simulink model "DUALportRAMinterface_v2"  (R2024a)
settings: Solver=FixedStepDiscrete  StartTime=0.0  StopTime=20  RelTol=1e-3
values from neighbouring files (symbols this model uses):
  Ts = 1/Fs    (= 7.50007500075e-06)    [new_generation_coeff.m]    (also in simon_test.m; simple_fft_test.m = 1/F; testPSD_c2d.m; testPSD_simulink.m)
undefined symbols (not defined in the file or in its folder): magnitude
libraries: hdlsllib x226, embmathops x6, simulink x1, hdlmdlgenlib x1, dsphdlxfrm2 x1
(part 1 of 5)
settings Model: DataTypeOverride=Off  Creator=Simon  LastModifiedBy=Simon
settings OptimizationCC: BlockReduction=off  ConditionallyExecuteInputs=off  DefaultParameterBehavior=Inlined  InheritOutputTypeSmallerThanSingle=on
settings DebuggingCC: AlgebraicLoopMsg=error  SingleTaskRateTransMsg=error  UnconnectedInputMsg=warning  UnconnectedOutputMsg=warning  UnconnectedLineMsg=warning
settings HardwareCC: ProdBitPerPointer=32  ProdBitPerSizeT=32  ProdBitPerPtrDiffT=32  ProdLargestAtomicFloat=None  ProdIntDivRoundTo=Undefined  ProdEndianess=Unspecified  ProdWordSize=32  ProdHWDeviceType=ASIC/FPGA->ASIC/FPGA  TargetBitPerPointer=64  TargetBitPerSizeT=64  TargetBitPerPtrDiffT=64  TargetLongLongMode=on  TargetIntDivRoundTo=Zero  TargetEndianess=LittleEndian  TargetWordSize=64  TargetHWDeviceType=Custom Processor->MATLAB Host Computer  ProdEqTarget=off

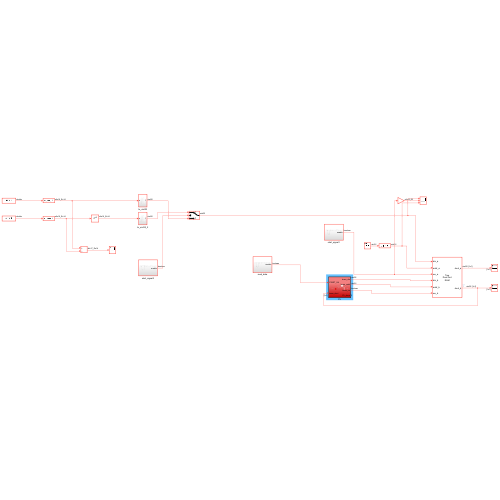
[thumbnail: Simulink's stored preview of the top-level diagram]
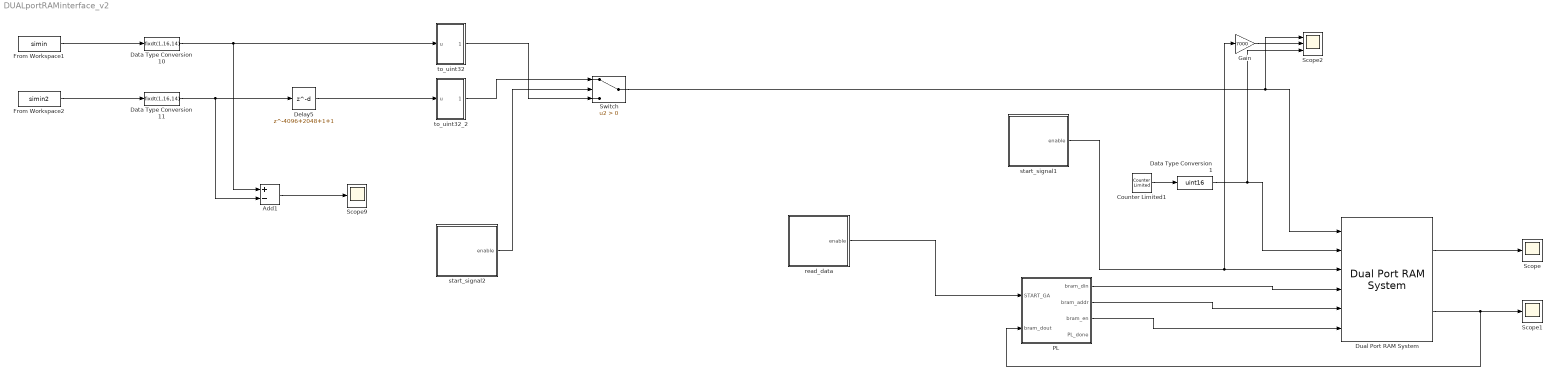
== system DUALportRAMinterface_v2 ==
  Add1 : Sum  Inputs=+-
  Counter Limited1 : simulink/Sources/Counter Limited  uplimit=14000  tsamp=Ts
  Data Type Conversion1 : DataTypeConversion  OutDataTypeStr=uint16  SaturateOnIntegerOverflow=off  RndMeth=Floor
  Data Type Conversion10 : DataTypeConversion  OutDataTypeStr=fixdt(1,16,14)  SaturateOnIntegerOverflow=off  RndMeth=Floor
  Data Type Conversion11 : DataTypeConversion  OutDataTypeStr=fixdt(1,16,14)  SaturateOnIntegerOverflow=off  RndMeth=Floor
  Delay5 : Delay  DelayLength=4096+2048+1+1  InitialCondition=0  SampleTime=Ts
  Dual Port RAM System : hdlsllib/HDL RAMs/Dual Port RAM System  RAMType=True dual port  AsyncRead=off  WriteOutputValue=New data  RAMInitialValue=0  allowBusInputs=off  WritesHaveOutput=on  NumReads=0  NumWrites=1  SimulateUsing=Code generation
  From Workspace1 : FromWorkspace  VariableName=simin  SampleTime=Ts
  From Workspace2 : FromWorkspace  VariableName=simin2  SampleTime=Ts
  Gain : Gain  Gain=7000
  PL : Subsystem
  Scope : Scope
  Scope1 : Scope
  Scope2 : Scope  NumInputPorts=3
  Scope9 : Scope
  Switch : Switch  Criteria=u2 > Threshold  SaturateOnIntegerOverflow=off  InputSameDT=off  OutDataTypeStr=Inherit: Same as first input
  read_data : Subsystem
  start_signal1 : Subsystem
  start_signal2 : Subsystem
  to_uint32 : Subsystem
  to_uint32_2 : Subsystem
  wires:
  Dual Port RAM System/1 -> Scope/1
  Counter Limited1/1 -> Data Type Conversion1/1
  Data Type Conversion1/1 -> Scope2/3, Dual Port RAM System/2
  start_signal1/1(enable) -> Dual Port RAM System/3, Gain/1
  PL/1(bram_din) -> Dual Port RAM System/4
  PL/2(bram_addr) -> Dual Port RAM System/5
  PL/3(bram_en) -> Dual Port RAM System/6
  Gain/1 -> Scope2/2
  read_data/1(enable) -> PL/1(START_GA)
  Dual Port RAM System/2 -> Scope1/1, PL/2(bram_dout)
  From Workspace1/1 -> Data Type Conversion10/1
  From Workspace2/1 -> Data Type Conversion11/1
  to_uint32/1(Out1) -> Switch/3
  to_uint32_2/1(Out1) -> Switch/1
  start_signal2/1(enable) -> Switch/2
  Delay5/1 -> to_uint32_2/1(u)
  Switch/1 -> Scope2/1, Dual Port RAM System/1
  Data Type Conversion11/1 -> Delay5/1, Add1/2
  Add1/1 -> Scope9/1
  Data Type Conversion10/1 -> Add1/1, to_uint32/1(u)

== system DUALportRAMinterface_v2/PL ==
  START_GA : Inport
  bram_dout : Inport  Port=2
  Bit Shift18 : hdlsllib/Logic and Bit Operations/Bit Shift  mode=Shift Right Logical  N=14
  Chart : Stateflow chart  TreatAsAtomicUnit=on
      settings: PortSchema="{\"entries\":[{\"content\":{\"sides\":[{\"content\":{\"connectorIds\":[\"In2\",\"In3\"]},\"type\":\"ConnectorPlacement.EquallySpacedRectSide\",\"uuid\":\"f3ce331f-c708-4668-a9cb-fb327ea74ab5\"},{\"content\":{\"connectorIds\":[\"Out1\",\"Out2\",\"Out3\"],\"side\":\"RIGHT\"},\"type\":\"ConnectorPlacement.EquallySpacedRectSide\",\"uuid\":\"3766927a-abff-497d-9544-2098881ba174\"},{\"content\":{\"side\":\"TOP\"},\"type\":\"ConnectorPlacement.EquallySpacedRectSide\",\"uuid\":\"ebfe3d64-ee7d-4953-a6ba-e7e40988decf\"},{\"content\":{\"connectorIds\":[\"In1\"],\"side\":\"BOTTOM\"},\"type\":\"ConnectorPlacement.EquallySpacedRectSide\",\"uuid\":\"f39ceaf8-4df7-4e40-9de5-da7597831fb4\"}]},\"type\":\"ConnectorPlacement.EquallySpacedConnector\",\"uuid\":\"89f60450-5933-42bb-b72b-5f8ec55483e0\"}],\"packageUris\":[\"http://schema.mathworks.com/mf0/Connector/R2020b\"],\"version\":\"1.0\"}"
  Data Type Conversion2 : DataTypeConversion  OutDataTypeStr=uint32  SaturateOnIntegerOverflow=off  RndMeth=Floor
  Data Type Conversion8 : DataTypeConversion  OutDataTypeStr=fixdt(0,30,14)  SaturateOnIntegerOverflow=off  RndMeth=Floor
  Data Type Conversion9 : DataTypeConversion  OutDataTypeStr=fixdt(1,16,14)  SaturateOnIntegerOverflow=off  RndMeth=Floor
  Delay : Delay  DelayLength=16  InitialCondition=0  SampleTime=Ts
  Demux : Demux  Outputs=7
  Multiport Switch : MultiPortSwitch  DataPortOrder=Specify indices  Inputs=8  DataPortIndices={0,1,2,3,4,5,6,7}  DataPortForDefault=Additional data port  DiagnosticForDefault=None  SaturateOnIntegerOverflow=off  InputSameDT=off
  index_counter : Subsystem
  integration_block1 : Subsystem
  to_uint32_1 : Subsystem
  to_uint32_2 : Subsystem
  to_uint32_3 : Subsystem
  to_uint32_4 : Subsystem
  to_uint32_5 : Subsystem
  to_uint32_6 : Subsystem
  bram_din : Outport
  bram_addr : Outport  Port=2
  bram_en : Outport  Port=3
  PL_done : Outport  Port=4
  wires:
  Multiport Switch/1 -> [PL_data]
  [counter_reset] -> index_counter/2(In2)
  index_counter/1(index_counter) -> Chart/3(counter), [address]
  [address] -> bram_addr/1
  [counter_increment] -> index_counter/1(In1)
  [address] -> Multiport Switch/1
  Chart/3(write_enable) -> [write_enable]
  integration_block1/1(ga_done) -> Delay/1, Chart/1(GA_done)
  START_GA/1 -> Chart/2(GPIO), integration_block1/3(start_ga)
  Chart/2(counter_reset) -> [counter_reset]
  Chart/1(counter_increment) -> [counter_increment]
  [PL_data] -> bram_din/1
  [write_enable] -> bram_en/1
  integration_block1/2(elite_individual) -> Demux/1
  Demux/1 -> Data Type Conversion2/1
  Demux/2 -> to_uint32_1/1(u_port)
  Demux/3 -> to_uint32_2/1(u_port)
  Demux/4 -> to_uint32_3/1(u_port)
  Demux/5 -> to_uint32_4/1(u_port)
  Demux/6 -> to_uint32_5/1(u_port)
  Demux/7 -> to_uint32_6/1(u_port)
  Data Type Conversion2/1 -> Multiport Switch/10, Multiport Switch/9, Multiport Switch/2
  to_uint32_1/1(Out1) -> Multiport Switch/3
  to_uint32_2/1(Out1) -> Multiport Switch/4
  to_uint32_3/1(Out1) -> Multiport Switch/5
  to_uint32_4/1(Out1) -> Multiport Switch/6
  to_uint32_5/1(Out1) -> Multiport Switch/7
  to_uint32_6/1(Out1) -> Multiport Switch/8
  Data Type Conversion9/1 -> integration_block1/1(data_in), integration_block1/2(data_in1)
  Bit Shift18/1 -> Data Type Conversion9/1
  Data Type Conversion8/1 -> Bit Shift18/1
  bram_dout/1 -> Data Type Conversion8/1
  [PL_done] -> PL_done/1
  Delay/1 -> [PL_done]

== system DUALportRAMinterface_v2/read_data ==
  Data Type Conversion29 : DataTypeConversion  OutDataTypeStr=boolean  SaturateOnIntegerOverflow=off  RndMeth=Floor
  Delay2 : Delay  DelayLength=1  InitialCondition=0  SampleTime=Ts
  Gain : Gain
  Step1 : Step  Time=Ts*14000  SampleTime=Ts
  XOR1 : Logic  Operator=XOR  IconShape=distinctive  AllPortsSameDT=off  OutDataTypeStr=boolean
  enable : Outport
  wires:
  XOR1/1 -> Gain/1
  Step1/1 -> Delay2/1, XOR1/1
  Delay2/1 -> XOR1/2
  Gain/1 -> Data Type Conversion29/1
  Data Type Conversion29/1 -> enable/1

== system DUALportRAMinterface_v2/start_signal1 ==
  Data Type Conversion29 : DataTypeConversion  OutDataTypeStr=boolean  SaturateOnIntegerOverflow=off  RndMeth=Floor
  Delay2 : Delay  DelayLength=(4096+2048+1+1)*2  InitialCondition=0  SampleTime=Ts
  Gain : Gain
  Step1 : Step  Time=Ts*0  SampleTime=Ts
  XOR1 : Logic  Operator=XOR  IconShape=distinctive  AllPortsSameDT=off  OutDataTypeStr=boolean
  enable : Outport
  wires:
  Data Type Conversion29/1 -> enable/1
  Gain/1 -> Data Type Conversion29/1
  Delay2/1 -> XOR1/2
  Step1/1 -> XOR1/1, Delay2/1
  XOR1/1 -> Gain/1

== system DUALportRAMinterface_v2/start_signal2 ==
  Data Type Conversion29 : DataTypeConversion  OutDataTypeStr=boolean  SaturateOnIntegerOverflow=off  RndMeth=Floor
  Delay2 : Delay  DelayLength=(4096+2048+1+1)*2  InitialCondition=0  SampleTime=Ts
  Gain : Gain
  Step1 : Step  Time=Ts*(4096+2048+1+1)  SampleTime=Ts
  XOR1 : Logic  Operator=XOR  IconShape=distinctive  AllPortsSameDT=off  OutDataTypeStr=boolean
  enable : Outport
  wires:
  XOR1/1 -> Gain/1
  Step1/1 -> Delay2/1, XOR1/1
  Delay2/1 -> XOR1/2
  Gain/1 -> Data Type Conversion29/1
  Data Type Conversion29/1 -> enable/1

== system DUALportRAMinterface_v2/to_uint32 ==
  u : Inport
  Bit Concat2 : hdlsllib/Logic and Bit Operations/Bit Concat  numInputs=16
  Bit Shift19 : hdlsllib/Logic and Bit Operations/Bit Shift  mode=Shift Left Logical  N=1
  Bit Shift20 : hdlsllib/Logic and Bit Operations/Bit Shift  mode=Shift Left Logical  N=10
  Bit Shift21 : hdlsllib/Logic and Bit Operations/Bit Shift  mode=Shift Right Logical  N=1
  Bit Shift22 : hdlsllib/Logic and Bit Operations/Bit Shift  mode=Shift Left Logical  N=11
  Bit Shift23 : hdlsllib/Logic and Bit Operations/Bit Shift  mode=Shift Left Logical  N=12
  Bit Shift24 : hdlsllib/Logic and Bit Operations/Bit Shift  mode=Shift Left Logical  N=13
  Bit Shift25 : hdlsllib/Logic and Bit Operations/Bit Shift  mode=Shift Left Logical  N=14
  Bit Shift26 : hdlsllib/Logic and Bit Operations/Bit Shift  mode=Shift Left Logical  N=2
  Bit Shift27 : hdlsllib/Logic and Bit Operations/Bit Shift  mode=Shift Left Logical  N=3
  Bit Shift28 : hdlsllib/Logic and Bit Operations/Bit Shift  mode=Shift Left Logical  N=4
  Bit Shift29 : hdlsllib/Logic and Bit Operations/Bit Shift  mode=Shift Left Logical  N=5
  Bit Shift30 : hdlsllib/Logic and Bit Operations/Bit Shift  mode=Shift Left Logical  N=6
  Bit Shift31 : hdlsllib/Logic and Bit Operations/Bit Shift  mode=Shift Left Logical  N=7
  Bit Shift32 : hdlsllib/Logic and Bit Operations/Bit Shift  mode=Shift Left Logical  N=8
  Bit Shift33 : hdlsllib/Logic and Bit Operations/Bit Shift  mode=Shift Left Logical  N=9
  Data Type Conversion{12..16,26,34..43} (16 alike) : DataTypeConversion  OutDataTypeStr=fixdt(0,1,0)  SaturateOnIntegerOverflow=off  RndMeth=Floor
  Data Type Conversion44 : DataTypeConversion  OutDataTypeStr=uint32  SaturateOnIntegerOverflow=off  RndMeth=Floor
  Out1 : Outport
  wires:
  Bit Shift22/1 -> Data Type Conversion40/1
  Bit Shift27/1 -> Data Type Conversion34/1
  Data Type Conversion36/1 -> Bit Concat2/3
  u/1 -> Bit Shift21/1, Data Type Conversion12/1, Bit Shift19/1, Bit Shift26/1, Bit Shift27/1, Bit Shift28/1, Bit Shift29/1, Bit Shift30/1, Bit Shift31/1, Bit Shift32/1, Bit Shift33/1, Bit Shift20/1, Bit Shift22/1, Bit Shift23/1, Bit Shift24/1, Bit Shift25/1
  Bit Shift20/1 -> Data Type Conversion41/1
  Data Type Conversion13/1 -> Bit Concat2/1
  Data Type Conversion40/1 -> Bit Concat2/13
  Bit Shift31/1 -> Data Type Conversion43/1
  Data Type Conversion26/1 -> Bit Concat2/6
  Data Type Conversion44/1 -> Out1/1
  Data Type Conversion35/1 -> Bit Concat2/4
  Data Type Conversion42/1 -> Bit Concat2/11
  Bit Shift19/1 -> Data Type Conversion36/1
  Data Type Conversion38/1 -> Bit Concat2/15
  Bit Shift25/1 -> Data Type Conversion37/1
  Data Type Conversion15/1 -> Bit Concat2/8
  Bit Shift30/1 -> Data Type Conversion15/1
  Data Type Conversion12/1 -> Bit Concat2/2
  Bit Shift32/1 -> Data Type Conversion14/1
  Data Type Conversion39/1 -> Bit Concat2/14
  Data Type Conversion34/1 -> Bit Concat2/5
  Data Type Conversion43/1 -> Bit Concat2/9
  Data Type Conversion16/1 -> Bit Concat2/7
  Bit Shift33/1 -> Data Type Conversion42/1
  Bit Shift24/1 -> Data Type Conversion38/1
  Data Type Conversion41/1 -> Bit Concat2/12
  Bit Shift23/1 -> Data Type Conversion39/1
  Bit Shift29/1 -> Data Type Conversion16/1
  Data Type Conversion37/1 -> Bit Concat2/16
  Bit Shift28/1 -> Data Type Conversion26/1
  Bit Shift21/1 -> Data Type Conversion13/1
  Bit Shift26/1 -> Data Type Conversion35/1
  Bit Concat2/1 -> Data Type Conversion44/1
  Data Type Conversion14/1 -> Bit Concat2/10

== system DUALportRAMinterface_v2/to_uint32_2 ==
  u : Inport
  Bit Concat2 : hdlsllib/Logic and Bit Operations/Bit Concat  numInputs=16
  Bit Shift19 : hdlsllib/Logic and Bit Operations/Bit Shift  mode=Shift Left Logical  N=1
  Bit Shift20 : hdlsllib/Logic and Bit Operations/Bit Shift  mode=Shift Left Logical  N=10
  Bit Shift21 : hdlsllib/Logic and Bit Operations/Bit Shift  mode=Shift Right Logical  N=1
  Bit Shift22 : hdlsllib/Logic and Bit Operations/Bit Shift  mode=Shift Left Logical  N=11
  Bit Shift23 : hdlsllib/Logic and Bit Operations/Bit Shift  mode=Shift Left Logical  N=12
  Bit Shift24 : hdlsllib/Logic and Bit Operations/Bit Shift  mode=Shift Left Logical  N=13
  Bit Shift25 : hdlsllib/Logic and Bit Operations/Bit Shift  mode=Shift Left Logical  N=14
  Bit Shift26 : hdlsllib/Logic and Bit Operations/Bit Shift  mode=Shift Left Logical  N=2
  Bit Shift27 : hdlsllib/Logic and Bit Operations/Bit Shift  mode=Shift Left Logical  N=3
  Bit Shift28 : hdlsllib/Logic and Bit Operations/Bit Shift  mode=Shift Left Logical  N=4
  Bit Shift29 : hdlsllib/Logic and Bit Operations/Bit Shift  mode=Shift Left Logical  N=5
  Bit Shift30 : hdlsllib/Logic and Bit Operations/Bit Shift  mode=Shift Left Logical  N=6
  Bit Shift31 : hdlsllib/Logic and Bit Operations/Bit Shift  mode=Shift Left Logical  N=7
  Bit Shift32 : hdlsllib/Logic and Bit Operations/Bit Shift  mode=Shift Left Logical  N=8
  Bit Shift33 : hdlsllib/Logic and Bit Operations/Bit Shift  mode=Shift Left Logical  N=9
  Data Type Conversion{12..16,26,34..43} (16 alike) : DataTypeConversion  OutDataTypeStr=fixdt(0,1,0)  SaturateOnIntegerOverflow=off  RndMeth=Floor
  Data Type Conversion44 : DataTypeConversion  OutDataTypeStr=uint32  SaturateOnIntegerOverflow=off  RndMeth=Floor
  Out1 : Outport
  wires:
  Data Type Conversion14/1 -> Bit Concat2/10
  Bit Concat2/1 -> Data Type Conversion44/1
  Bit Shift26/1 -> Data Type Conversion35/1
  Bit Shift21/1 -> Data Type Conversion13/1
  Bit Shift28/1 -> Data Type Conversion26/1
  Data Type Conversion37/1 -> Bit Concat2/16
  Bit Shift29/1 -> Data Type Conversion16/1
  Bit Shift23/1 -> Data Type Conversion39/1
  Data Type Conversion41/1 -> Bit Concat2/12
  Bit Shift24/1 -> Data Type Conversion38/1
  Bit Shift33/1 -> Data Type Conversion42/1
  Data Type Conversion16/1 -> Bit Concat2/7
  Data Type Conversion43/1 -> Bit Concat2/9
  Data Type Conversion34/1 -> Bit Concat2/5
  Data Type Conversion39/1 -> Bit Concat2/14
  Bit Shift32/1 -> Data Type Conversion14/1
  Data Type Conversion12/1 -> Bit Concat2/2
  Bit Shift30/1 -> Data Type Conversion15/1
  Data Type Conversion15/1 -> Bit Concat2/8
  Bit Shift25/1 -> Data Type Conversion37/1
  Data Type Conversion38/1 -> Bit Concat2/15
  Bit Shift19/1 -> Data Type Conversion36/1
  Data Type Conversion42/1 -> Bit Concat2/11
  Data Type Conversion35/1 -> Bit Concat2/4
  Data Type Conversion44/1 -> Out1/1
  Data Type Conversion26/1 -> Bit Concat2/6
  Bit Shift31/1 -> Data Type Conversion43/1
  Data Type Conversion40/1 -> Bit Concat2/13
  Data Type Conversion13/1 -> Bit Concat2/1
  Bit Shift20/1 -> Data Type Conversion41/1
  u/1 -> Bit Shift25/1, Bit Shift24/1, Bit Shift23/1, Bit Shift22/1, Bit Shift20/1, Bit Shift33/1, Bit Shift32/1, Bit Shift31/1, Bit Shift30/1, Bit Shift29/1, Bit Shift28/1, Bit Shift27/1, Bit Shift26/1, Bit Shift19/1, Data Type Conversion12/1, Bit Shift21/1
  Data Type Conversion36/1 -> Bit Concat2/3
  Bit Shift27/1 -> Data Type Conversion34/1
  Bit Shift22/1 -> Data Type Conversion40/1

== system DUALportRAMinterface_v2/PL/index_counter ==
  In1 : Inport
  In2 : Inport  Port=2
  Add : Sum  OutDataTypeStr=Inherit: Same as first input
  Constant18 : Constant  OutDataTypeStr=fixdt(0,16,0)  SampleTime=Ts
  Constant19 : Constant  Value=0  OutDataTypeStr=fixdt(0,16,0)  SampleTime=Ts
  Constant20 : Constant  Value=0  OutDataTypeStr=uint16  SampleTime=Ts
  Delay : Delay  DelayLength=1  InitialCondition=0  SampleTime=Ts
  Switch : Switch  Criteria=u2 > Threshold  SaturateOnIntegerOverflow=off  InputSameDT=off  OutDataTypeStr=Inherit: Same as first input
  Switch8 : Switch  Criteria=u2 > Threshold  SaturateOnIntegerOverflow=off  InputSameDT=off  OutDataTypeStr=Inherit: Same as first input
  index_counter : Outport
  wires:
  Constant19/1 -> Switch/3
  Switch8/1 -> Add/2
  Switch/1 -> Add/1
  Delay/1 -> index_counter/1, Switch8/3
  In2/1 -> Switch8/2
  Add/1 -> Delay/1
  Constant20/1 -> Switch8/1
  Constant18/1 -> Switch/1
  In1/1 -> Switch/2

== system DUALportRAMinterface_v2/PL/integration_block1 ==
  data_in : Inport
  data_in1 : Inport  Port=2
  start_ga : Inport  Port=3
  D2 : Subsystem
      settings: PortSchema="{\"entries\":[{\"content\":{\"sides\":[{\"content\":{\"connectorIds\":[\"In1\",\"In2\"]},\"type\":\"ConnectorPlacement.EquallySpacedRectSide\",\"uuid\":\"5abe48ab-1b34-4cb0-8d41-07cb17904e64\"},{\"content\":{\"connectorIds\":[\"Out1\"],\"side\":\"RIGHT\"},\"type\":\"ConnectorPlacement.EquallySpacedRectSide\",\"uuid\":\"19bc24ff-88f3-42df-af8e-ecb9c1c6119c\"},{\"content\":{\"connectorIds\":[\"In3\"],\"side\":\"TOP\"},\"type\":\"ConnectorPlacement.EquallySpacedRectSide\",\"uuid\":\"46fc65c4-6cee-4e0a-9107-9d106d0a52a5\"},{\"content\":{\"connectorIds\":[\"In4\"],\"side\":\"BOTTOM\"},\"type\":\"ConnectorPlacement.EquallySpacedRectSide\",\"uuid\":\"10a5fc09-3948-4556-8b0c-050853396926\"}]},\"type\":\"ConnectorPlacement.EquallySpacedConnector\",\"uuid\":\"9cc35bfe-5b00-42b0-9811-425d4f0f8f7b\"}],\"packageUris\":[\"http://schema.mathworks.com/mf0/Connector/R2020b\"],\"version\":\"1.0\"}"
  Delay : Delay  DelayLength=6145  InitialCondition=0  UseCircularBuffer=on  SampleTime=Ts
  Delay3 : Delay  DelayLength=1  InitialCondition=0  SampleTime=Ts
  FFT : dsphdlxfrm2/FFT  Architecture=Burst Radix 2  FFTLengthSource=Property  FFTLength=4096  FFTLengthMax=1024  ComplexMultiplication=Use 4 multipliers and 2 adders  BitReversedOutput=off  BitReversedInput=off  Normalize=off  SimulateUsing=Code generation  RoundingMethod=Floor  ResetInputPort=on  StartOutputPort=off  EndOutputPort=off
  FIFO_system1 : Subsystem
  FIFO_system3 : Subsystem
  GA_main : Subsystem
      settings: PortSchema="{\"entries\":[{\"content\":{\"sides\":[{\"content\":{\"connectorIds\":[\"In1\",\"In2\",\"In3\",\"In4\",\"In5\",\"In6\",\"In7\",\"In8\",\"In9\",\"In10\",\"In11\"]},\"type\":\"ConnectorPlacement.EquallySpacedRectSide\",\"uuid\":\"daccc056-a93f-45e5-9369-71b73e32651e\"},{\"content\":{\"connectorIds\":[\"Out1\",\"Out2\"],\"side\":\"RIGHT\"},\"type\":\"ConnectorPlacement.EquallySpacedRectSide\",\"uuid\":\"82109161-9ebe-455f-914b-56f9927b10eb\"},{\"content\":{\"connectorIds\":[\"Out3\",\"Out4\",\"Out5\",\"In12\",\"In13\"],\"side\":\"TOP\"},\"type\":\"ConnectorPlacement.EquallySpacedRectSide\",\"uuid\":\"07b2e20b-bb92-4769-b746-3d44a115cdd8\"}]},\"type\":\"ConnectorPlacement.EquallySpacedConnector\",\"uuid\":\"c9f522d4-4f80-4900-b8a5-3110692e6ae8\"}],\"packageUris\":[\"http://schema.mathworks.com/mf0/Connector/R2020b\"],\"version\":\"1.0\"}"
  Scope1 : Scope
  Subsystem : Subsystem
  Sum : Sum  Inputs=|+-  OutDataTypeStr=Inherit: Same as first input
  Terminator : Terminator
  Terminator1 : Terminator
  Terminator2 : Terminator
  accumulator_scorer : Subsystem
  ga_done : Outport
  elite_individual : Outport  Port=2
  wires:
  FFT/2 -> accumulator_scorer/2(valid_fft)
  FIFO_system3/2(data_valid) -> Terminator1/1
  accumulator_scorer/1(individual_score) -> GA_main/2(score_result), Scope1/1
  FIFO_system1/1(data_out) -> Sum/1
  start_ga/1 -> GA_main/1(start_ga), Subsystem/1(enable)
  D2/1(response) -> Sum/2
  FFT/1 -> accumulator_scorer/1(data_in)
  FFT/3 -> Terminator/1
  GA_main/5(load_fifo) -> FIFO_system1/3(load_fifo)
  GA_main/4(FIFO_out_en) -> D2/2(push_individual), FIFO_system3/2(enable_output), FIFO_system1/2(enable_output)
  data_in/1 -> FIFO_system1/1(data_in)
  GA_main/2(ga_done) -> ga_done/1
  FIFO_system3/1(data_out) -> D2/1(GAerror)
  GA_main/3(individual_to_d2) -> D2/4(Individual_input)
  accumulator_scorer/2(individual_score_valid) -> Delay3/1
  FIFO_system3/3(reset_fft) -> Terminator2/1
  Delay3/1 -> GA_main/13(score_done)
  data_in1/1 -> FIFO_system3/1(data_in)
  FIFO_system1/2(data_valid) -> FFT/2
  FIFO_system1/3(reset_fft) -> Delay/1, FFT/3
  FIFO_system3/4(FIFO_full) -> GA_main/12(FIFO_full)
  Sum/1 -> FFT/1
  Delay/1 -> D2/3(reset_D2)
  Subsystem/1(random_gene_out) -> GA_main/3(random_gene)
  Subsystem/2(random_method_out) -> GA_main/4(random_method)
  Subsystem/3(b2_random_out) -> GA_main/5(b2rnd)
  Subsystem/4(b3_random_out) -> GA_main/6(b3rnd)
  Subsystem/5(b4_random_out) -> GA_main/7(b4rnd)
  Subsystem/6(a2_random_out) -> GA_main/8(a2rnd)
  Subsystem/7(a3_random_out) -> GA_main/9(a3rnd)
  Subsystem/8(a4_random_out) -> GA_main/10(a4rnd)
  Subsystem/9(random_sample_out) -> GA_main/11(tb_random_sample)
  FIFO_system1/4(FIFO_full) -> FIFO_system3/3(load_fifo)
  GA_main/1(elite_individual) -> elite_individual/1

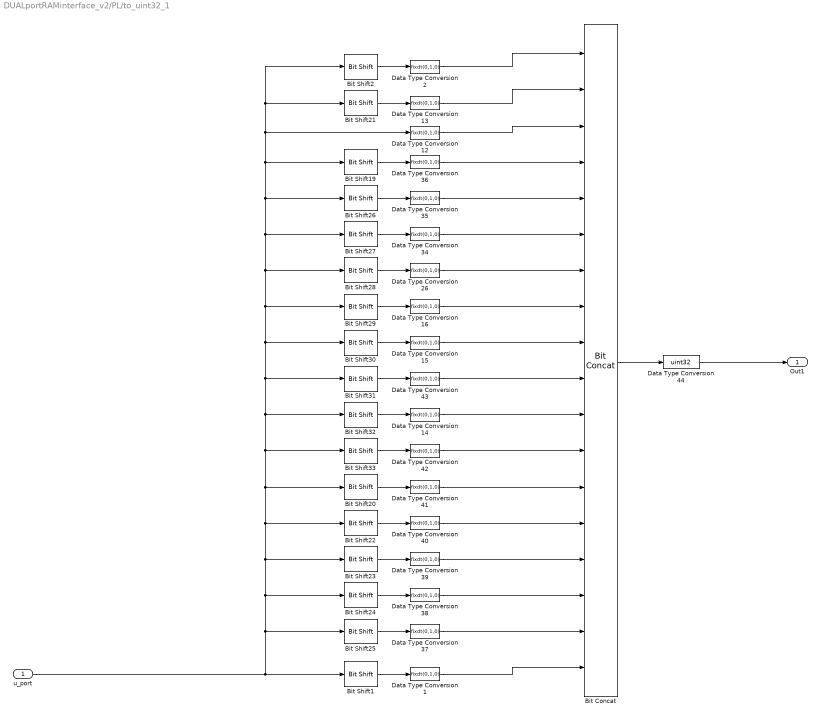
== system DUALportRAMinterface_v2/PL/to_uint32_1 ==
  u_port : Inport
  Bit Concat : hdlsllib/Logic and Bit Operations/Bit Concat  numInputs=18
  Bit Shift1 : hdlsllib/Logic and Bit Operations/Bit Shift  mode=Shift Left Logical  N=15
  Bit Shift19 : hdlsllib/Logic and Bit Operations/Bit Shift  mode=Shift Left Logical  N=1
  Bit Shift2 : hdlsllib/Logic and Bit Operations/Bit Shift  mode=Shift Right Logical  N=16
  Bit Shift20 : hdlsllib/Logic and Bit Operations/Bit Shift  mode=Shift Left Logical  N=10
  Bit Shift21 : hdlsllib/Logic and Bit Operations/Bit Shift  mode=Shift Right Logical  N=1
  Bit Shift22 : hdlsllib/Logic and Bit Operations/Bit Shift  mode=Shift Left Logical  N=11
  Bit Shift23 : hdlsllib/Logic and Bit Operations/Bit Shift  mode=Shift Left Logical  N=12
  Bit Shift24 : hdlsllib/Logic and Bit Operations/Bit Shift  mode=Shift Left Logical  N=13
  Bit Shift25 : hdlsllib/Logic and Bit Operations/Bit Shift  mode=Shift Left Logical  N=14
  Bit Shift26 : hdlsllib/Logic and Bit Operations/Bit Shift  mode=Shift Left Logical  N=2
  Bit Shift27 : hdlsllib/Logic and Bit Operations/Bit Shift  mode=Shift Left Logical  N=3
  Bit Shift28 : hdlsllib/Logic and Bit Operations/Bit Shift  mode=Shift Left Logical  N=4
  Bit Shift29 : hdlsllib/Logic and Bit Operations/Bit Shift  mode=Shift Left Logical  N=5
  Bit Shift30 : hdlsllib/Logic and Bit Operations/Bit Shift  mode=Shift Left Logical  N=6
  Bit Shift31 : hdlsllib/Logic and Bit Operations/Bit Shift  mode=Shift Left Logical  N=7
  Bit Shift32 : hdlsllib/Logic and Bit Operations/Bit Shift  mode=Shift Left Logical  N=8
  Bit Shift33 : hdlsllib/Logic and Bit Operations/Bit Shift  mode=Shift Left Logical  N=9
  Data Type Conversion{1..2,12..16,26,34..43} (18 alike) : DataTypeConversion  OutDataTypeStr=fixdt(0,1,0)  SaturateOnIntegerOverflow=off  RndMeth=Floor
  Data Type Conversion44 : DataTypeConversion  OutDataTypeStr=uint32  SaturateOnIntegerOverflow=off  RndMeth=Floor
  Out1 : Outport
  wires:
  Data Type Conversion44/1 -> Out1/1
  Data Type Conversion42/1 -> Bit Concat/12
  Bit Shift32/1 -> Data Type Conversion14/1
  Data Type Conversion40/1 -> Bit Concat/14
  Data Type Conversion37/1 -> Bit Concat/17
  Data Type Conversion38/1 -> Bit Concat/16
  Bit Shift30/1 -> Data Type Conversion15/1
  Data Type Conversion13/1 -> Bit Concat/2
  Bit Shift19/1 -> Data Type Conversion36/1
  Data Type Conversion16/1 -> Bit Concat/8
  Data Type Conversion35/1 -> Bit Concat/5
  Bit Shift1/1 -> Data Type Conversion1/1
  Bit Shift24/1 -> Data Type Conversion38/1
  Data Type Conversion36/1 -> Bit Concat/4
  Bit Shift28/1 -> Data Type Conversion26/1
  Data Type Conversion34/1 -> Bit Concat/6
  Bit Shift26/1 -> Data Type Conversion35/1
  Bit Shift29/1 -> Data Type Conversion16/1
  Bit Shift2/1 -> Data Type Conversion2/1
  Data Type Conversion41/1 -> Bit Concat/13
  Bit Shift25/1 -> Data Type Conversion37/1
  Bit Shift23/1 -> Data Type Conversion39/1
  Bit Shift33/1 -> Data Type Conversion42/1
  Data Type Conversion43/1 -> Bit Concat/10
  Data Type Conversion15/1 -> Bit Concat/9
  Data Type Conversion39/1 -> Bit Concat/15
  Bit Shift31/1 -> Data Type Conversion43/1
  Bit Shift20/1 -> Data Type Conversion41/1
  Bit Shift22/1 -> Data Type Conversion40/1
  Bit Shift27/1 -> Data Type Conversion34/1
  Data Type Conversion12/1 -> Bit Concat/3
  Bit Shift21/1 -> Data Type Conversion13/1
  Data Type Conversion26/1 -> Bit Concat/7
  Data Type Conversion2/1 -> Bit Concat/1
  Data Type Conversion1/1 -> Bit Concat/18
  Data Type Conversion14/1 -> Bit Concat/11
  u_port/1 -> Bit Shift25/1, Bit Shift24/1, Bit Shift23/1, Bit Shift22/1, Bit Shift20/1, Bit Shift33/1, Bit Shift32/1, Bit Shift31/1, Bit Shift30/1, Bit Shift29/1, Bit Shift28/1, Bit Shift27/1, Bit Shift26/1, Bit Shift19/1, Data Type Conversion12/1, Bit Shift2/1, Bit Shift21/1, Bit Shift1/1
  Bit Concat/1 -> Data Type Conversion44/1

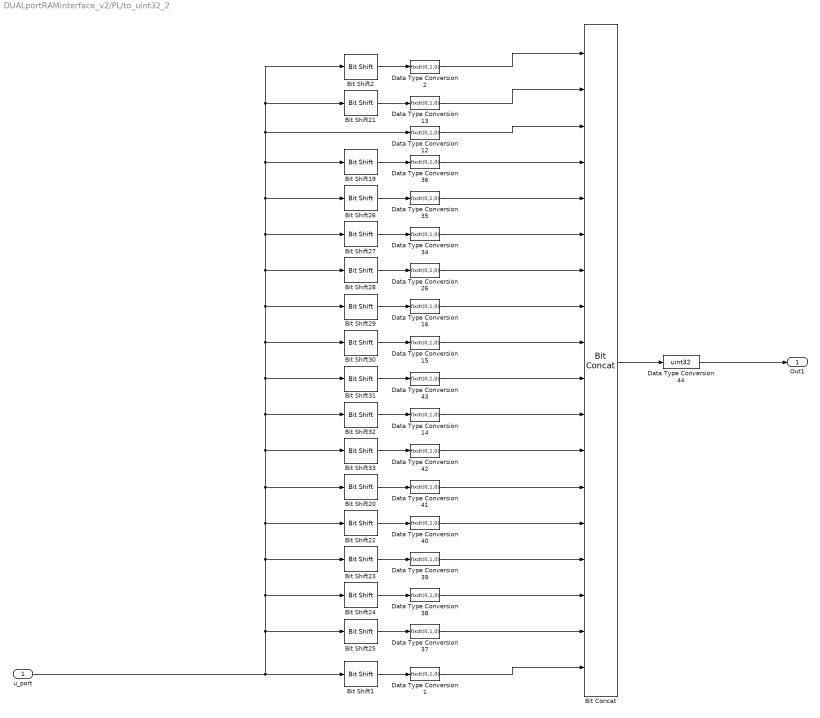
== system DUALportRAMinterface_v2/PL/to_uint32_2 ==
  u_port : Inport
  Bit Concat : hdlsllib/Logic and Bit Operations/Bit Concat  numInputs=18
  Bit Shift1 : hdlsllib/Logic and Bit Operations/Bit Shift  mode=Shift Left Logical  N=15
  Bit Shift19 : hdlsllib/Logic and Bit Operations/Bit Shift  mode=Shift Left Logical  N=1
  Bit Shift2 : hdlsllib/Logic and Bit Operations/Bit Shift  mode=Shift Right Logical  N=16
  Bit Shift20 : hdlsllib/Logic and Bit Operations/Bit Shift  mode=Shift Left Logical  N=10
  Bit Shift21 : hdlsllib/Logic and Bit Operations/Bit Shift  mode=Shift Right Logical  N=1
  Bit Shift22 : hdlsllib/Logic and Bit Operations/Bit Shift  mode=Shift Left Logical  N=11
  Bit Shift23 : hdlsllib/Logic and Bit Operations/Bit Shift  mode=Shift Left Logical  N=12
  Bit Shift24 : hdlsllib/Logic and Bit Operations/Bit Shift  mode=Shift Left Logical  N=13
  Bit Shift25 : hdlsllib/Logic and Bit Operations/Bit Shift  mode=Shift Left Logical  N=14
  Bit Shift26 : hdlsllib/Logic and Bit Operations/Bit Shift  mode=Shift Left Logical  N=2
  Bit Shift27 : hdlsllib/Logic and Bit Operations/Bit Shift  mode=Shift Left Logical  N=3
  Bit Shift28 : hdlsllib/Logic and Bit Operations/Bit Shift  mode=Shift Left Logical  N=4
  Bit Shift29 : hdlsllib/Logic and Bit Operations/Bit Shift  mode=Shift Left Logical  N=5
  Bit Shift30 : hdlsllib/Logic and Bit Operations/Bit Shift  mode=Shift Left Logical  N=6
  Bit Shift31 : hdlsllib/Logic and Bit Operations/Bit Shift  mode=Shift Left Logical  N=7
  Bit Shift32 : hdlsllib/Logic and Bit Operations/Bit Shift  mode=Shift Left Logical  N=8
  Bit Shift33 : hdlsllib/Logic and Bit Operations/Bit Shift  mode=Shift Left Logical  N=9
  Data Type Conversion{1..2,12..16,26,34..43} (18 alike) : DataTypeConversion  OutDataTypeStr=fixdt(0,1,0)  SaturateOnIntegerOverflow=off  RndMeth=Floor
  Data Type Conversion44 : DataTypeConversion  OutDataTypeStr=uint32  SaturateOnIntegerOverflow=off  RndMeth=Floor
  Out1 : Outport
  wires:
  Bit Concat/1 -> Data Type Conversion44/1
  u_port/1 -> Bit Shift1/1, Bit Shift21/1, Bit Shift2/1, Data Type Conversion12/1, Bit Shift19/1, Bit Shift26/1, Bit Shift27/1, Bit Shift28/1, Bit Shift29/1, Bit Shift30/1, Bit Shift31/1, Bit Shift32/1, Bit Shift33/1, Bit Shift20/1, Bit Shift22/1, Bit Shift23/1, Bit Shift24/1, Bit Shift25/1
  Data Type Conversion14/1 -> Bit Concat/11
  Data Type Conversion1/1 -> Bit Concat/18
  Data Type Conversion2/1 -> Bit Concat/1
  Data Type Conversion26/1 -> Bit Concat/7
  Bit Shift21/1 -> Data Type Conversion13/1
  Data Type Conversion12/1 -> Bit Concat/3
  Bit Shift27/1 -> Data Type Conversion34/1
  Bit Shift22/1 -> Data Type Conversion40/1
  Bit Shift20/1 -> Data Type Conversion41/1
  Bit Shift31/1 -> Data Type Conversion43/1
  Data Type Conversion39/1 -> Bit Concat/15
  Data Type Conversion15/1 -> Bit Concat/9
  Data Type Conversion43/1 -> Bit Concat/10
  Bit Shift33/1 -> Data Type Conversion42/1
  Bit Shift23/1 -> Data Type Conversion39/1
  Bit Shift25/1 -> Data Type Conversion37/1
  Data Type Conversion41/1 -> Bit Concat/13
  Bit Shift2/1 -> Data Type Conversion2/1
  Bit Shift29/1 -> Data Type Conversion16/1
  Bit Shift26/1 -> Data Type Conversion35/1
  Data Type Conversion34/1 -> Bit Concat/6
  Bit Shift28/1 -> Data Type Conversion26/1
  Data Type Conversion36/1 -> Bit Concat/4
  Bit Shift24/1 -> Data Type Conversion38/1
  Bit Shift1/1 -> Data Type Conversion1/1
  Data Type Conversion35/1 -> Bit Concat/5
  Data Type Conversion16/1 -> Bit Concat/8
  Bit Shift19/1 -> Data Type Conversion36/1
  Data Type Conversion13/1 -> Bit Concat/2
  Bit Shift30/1 -> Data Type Conversion15/1
  Data Type Conversion38/1 -> Bit Concat/16
  Data Type Conversion37/1 -> Bit Concat/17
  Data Type Conversion40/1 -> Bit Concat/14
  Bit Shift32/1 -> Data Type Conversion14/1
  Data Type Conversion42/1 -> Bit Concat/12
  Data Type Conversion44/1 -> Out1/1

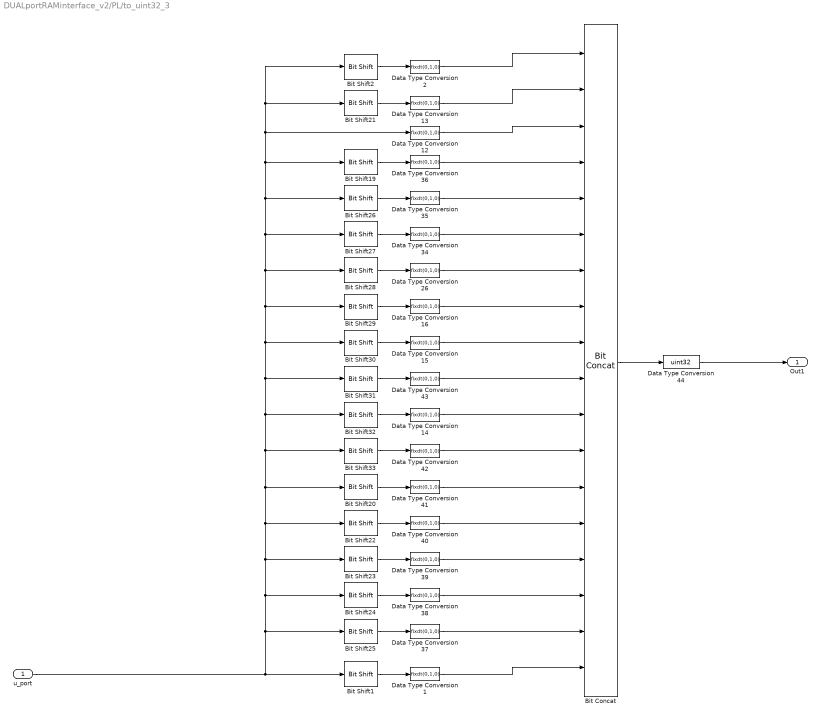
== system DUALportRAMinterface_v2/PL/to_uint32_3 ==
  u_port : Inport
  Bit Concat : hdlsllib/Logic and Bit Operations/Bit Concat  numInputs=18
  Bit Shift1 : hdlsllib/Logic and Bit Operations/Bit Shift  mode=Shift Left Logical  N=15
  Bit Shift19 : hdlsllib/Logic and Bit Operations/Bit Shift  mode=Shift Left Logical  N=1
  Bit Shift2 : hdlsllib/Logic and Bit Operations/Bit Shift  mode=Shift Right Logical  N=16
  Bit Shift20 : hdlsllib/Logic and Bit Operations/Bit Shift  mode=Shift Left Logical  N=10
  Bit Shift21 : hdlsllib/Logic and Bit Operations/Bit Shift  mode=Shift Right Logical  N=1
  Bit Shift22 : hdlsllib/Logic and Bit Operations/Bit Shift  mode=Shift Left Logical  N=11
  Bit Shift23 : hdlsllib/Logic and Bit Operations/Bit Shift  mode=Shift Left Logical  N=12
  Bit Shift24 : hdlsllib/Logic and Bit Operations/Bit Shift  mode=Shift Left Logical  N=13
  Bit Shift25 : hdlsllib/Logic and Bit Operations/Bit Shift  mode=Shift Left Logical  N=14
  Bit Shift26 : hdlsllib/Logic and Bit Operations/Bit Shift  mode=Shift Left Logical  N=2
  Bit Shift27 : hdlsllib/Logic and Bit Operations/Bit Shift  mode=Shift Left Logical  N=3
  Bit Shift28 : hdlsllib/Logic and Bit Operations/Bit Shift  mode=Shift Left Logical  N=4
  Bit Shift29 : hdlsllib/Logic and Bit Operations/Bit Shift  mode=Shift Left Logical  N=5
  Bit Shift30 : hdlsllib/Logic and Bit Operations/Bit Shift  mode=Shift Left Logical  N=6
  Bit Shift31 : hdlsllib/Logic and Bit Operations/Bit Shift  mode=Shift Left Logical  N=7
  Bit Shift32 : hdlsllib/Logic and Bit Operations/Bit Shift  mode=Shift Left Logical  N=8
  Bit Shift33 : hdlsllib/Logic and Bit Operations/Bit Shift  mode=Shift Left Logical  N=9
  Data Type Conversion{1..2,12..16,26,34..43} (18 alike) : DataTypeConversion  OutDataTypeStr=fixdt(0,1,0)  SaturateOnIntegerOverflow=off  RndMeth=Floor
  Data Type Conversion44 : DataTypeConversion  OutDataTypeStr=uint32  SaturateOnIntegerOverflow=off  RndMeth=Floor
  Out1 : Outport
  wires:
  Data Type Conversion44/1 -> Out1/1
  Data Type Conversion42/1 -> Bit Concat/12
  Bit Shift32/1 -> Data Type Conversion14/1
  Data Type Conversion40/1 -> Bit Concat/14
  Data Type Conversion37/1 -> Bit Concat/17
  Data Type Conversion38/1 -> Bit Concat/16
  Bit Shift30/1 -> Data Type Conversion15/1
  Data Type Conversion13/1 -> Bit Concat/2
  Bit Shift19/1 -> Data Type Conversion36/1
  Data Type Conversion16/1 -> Bit Concat/8
  Data Type Conversion35/1 -> Bit Concat/5
  Bit Shift1/1 -> Data Type Conversion1/1
  Bit Shift24/1 -> Data Type Conversion38/1
  Data Type Conversion36/1 -> Bit Concat/4
  Bit Shift28/1 -> Data Type Conversion26/1
  Data Type Conversion34/1 -> Bit Concat/6
  Bit Shift26/1 -> Data Type Conversion35/1
  Bit Shift29/1 -> Data Type Conversion16/1
  Bit Shift2/1 -> Data Type Conversion2/1
  Data Type Conversion41/1 -> Bit Concat/13
  Bit Shift25/1 -> Data Type Conversion37/1
  Bit Shift23/1 -> Data Type Conversion39/1
  Bit Shift33/1 -> Data Type Conversion42/1
  Data Type Conversion43/1 -> Bit Concat/10
  Data Type Conversion15/1 -> Bit Concat/9
  Data Type Conversion39/1 -> Bit Concat/15
  Bit Shift31/1 -> Data Type Conversion43/1
  Bit Shift20/1 -> Data Type Conversion41/1
  Bit Shift22/1 -> Data Type Conversion40/1
  Bit Shift27/1 -> Data Type Conversion34/1
  Data Type Conversion12/1 -> Bit Concat/3
  Bit Shift21/1 -> Data Type Conversion13/1
  Data Type Conversion26/1 -> Bit Concat/7
  Data Type Conversion2/1 -> Bit Concat/1
  Data Type Conversion1/1 -> Bit Concat/18
  Data Type Conversion14/1 -> Bit Concat/11
  u_port/1 -> Bit Shift25/1, Bit Shift24/1, Bit Shift23/1, Bit Shift22/1, Bit Shift20/1, Bit Shift33/1, Bit Shift32/1, Bit Shift31/1, Bit Shift30/1, Bit Shift29/1, Bit Shift28/1, Bit Shift27/1, Bit Shift26/1, Bit Shift19/1, Data Type Conversion12/1, Bit Shift2/1, Bit Shift21/1, Bit Shift1/1
  Bit Concat/1 -> Data Type Conversion44/1

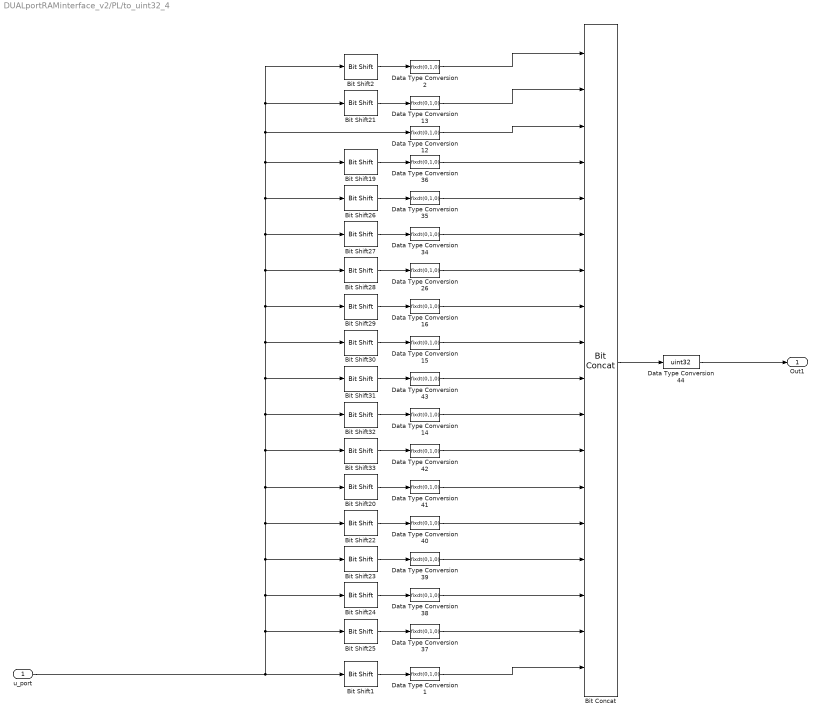
== system DUALportRAMinterface_v2/PL/to_uint32_4 ==
  u_port : Inport
  Bit Concat : hdlsllib/Logic and Bit Operations/Bit Concat  numInputs=18
  Bit Shift1 : hdlsllib/Logic and Bit Operations/Bit Shift  mode=Shift Left Logical  N=15
  Bit Shift19 : hdlsllib/Logic and Bit Operations/Bit Shift  mode=Shift Left Logical  N=1
  Bit Shift2 : hdlsllib/Logic and Bit Operations/Bit Shift  mode=Shift Right Logical  N=16
  Bit Shift20 : hdlsllib/Logic and Bit Operations/Bit Shift  mode=Shift Left Logical  N=10
  Bit Shift21 : hdlsllib/Logic and Bit Operations/Bit Shift  mode=Shift Right Logical  N=1
  Bit Shift22 : hdlsllib/Logic and Bit Operations/Bit Shift  mode=Shift Left Logical  N=11
  Bit Shift23 : hdlsllib/Logic and Bit Operations/Bit Shift  mode=Shift Left Logical  N=12
  Bit Shift24 : hdlsllib/Logic and Bit Operations/Bit Shift  mode=Shift Left Logical  N=13
  Bit Shift25 : hdlsllib/Logic and Bit Operations/Bit Shift  mode=Shift Left Logical  N=14
  Bit Shift26 : hdlsllib/Logic and Bit Operations/Bit Shift  mode=Shift Left Logical  N=2
  Bit Shift27 : hdlsllib/Logic and Bit Operations/Bit Shift  mode=Shift Left Logical  N=3
  Bit Shift28 : hdlsllib/Logic and Bit Operations/Bit Shift  mode=Shift Left Logical  N=4
  Bit Shift29 : hdlsllib/Logic and Bit Operations/Bit Shift  mode=Shift Left Logical  N=5
  Bit Shift30 : hdlsllib/Logic and Bit Operations/Bit Shift  mode=Shift Left Logical  N=6
  Bit Shift31 : hdlsllib/Logic and Bit Operations/Bit Shift  mode=Shift Left Logical  N=7
  Bit Shift32 : hdlsllib/Logic and Bit Operations/Bit Shift  mode=Shift Left Logical  N=8
  Bit Shift33 : hdlsllib/Logic and Bit Operations/Bit Shift  mode=Shift Left Logical  N=9
  Data Type Conversion{1..2,12..16,26,34..43} (18 alike) : DataTypeConversion  OutDataTypeStr=fixdt(0,1,0)  SaturateOnIntegerOverflow=off  RndMeth=Floor
  Data Type Conversion44 : DataTypeConversion  OutDataTypeStr=uint32  SaturateOnIntegerOverflow=off  RndMeth=Floor
  Out1 : Outport
  wires:
  Bit Concat/1 -> Data Type Conversion44/1
  u_port/1 -> Bit Shift1/1, Bit Shift21/1, Bit Shift2/1, Data Type Conversion12/1, Bit Shift19/1, Bit Shift26/1, Bit Shift27/1, Bit Shift28/1, Bit Shift29/1, Bit Shift30/1, Bit Shift31/1, Bit Shift32/1, Bit Shift33/1, Bit Shift20/1, Bit Shift22/1, Bit Shift23/1, Bit Shift24/1, Bit Shift25/1
  Data Type Conversion14/1 -> Bit Concat/11
  Data Type Conversion1/1 -> Bit Concat/18
  Data Type Conversion2/1 -> Bit Concat/1
  Data Type Conversion26/1 -> Bit Concat/7
  Bit Shift21/1 -> Data Type Conversion13/1
  Data Type Conversion12/1 -> Bit Concat/3
  Bit Shift27/1 -> Data Type Conversion34/1
  Bit Shift22/1 -> Data Type Conversion40/1
  Bit Shift20/1 -> Data Type Conversion41/1
  Bit Shift31/1 -> Data Type Conversion43/1
  Data Type Conversion39/1 -> Bit Concat/15
  Data Type Conversion15/1 -> Bit Concat/9
  Data Type Conversion43/1 -> Bit Concat/10
  Bit Shift33/1 -> Data Type Conversion42/1
  Bit Shift23/1 -> Data Type Conversion39/1
  Bit Shift25/1 -> Data Type Conversion37/1
  Data Type Conversion41/1 -> Bit Concat/13
  Bit Shift2/1 -> Data Type Conversion2/1
  Bit Shift29/1 -> Data Type Conversion16/1
  Bit Shift26/1 -> Data Type Conversion35/1
  Data Type Conversion34/1 -> Bit Concat/6
  Bit Shift28/1 -> Data Type Conversion26/1
  Data Type Conversion36/1 -> Bit Concat/4
  Bit Shift24/1 -> Data Type Conversion38/1
  Bit Shift1/1 -> Data Type Conversion1/1
  Data Type Conversion35/1 -> Bit Concat/5
  Data Type Conversion16/1 -> Bit Concat/8
  Bit Shift19/1 -> Data Type Conversion36/1
  Data Type Conversion13/1 -> Bit Concat/2
  Bit Shift30/1 -> Data Type Conversion15/1
  Data Type Conversion38/1 -> Bit Concat/16
  Data Type Conversion37/1 -> Bit Concat/17
  Data Type Conversion40/1 -> Bit Concat/14
  Bit Shift32/1 -> Data Type Conversion14/1
  Data Type Conversion42/1 -> Bit Concat/12
  Data Type Conversion44/1 -> Out1/1

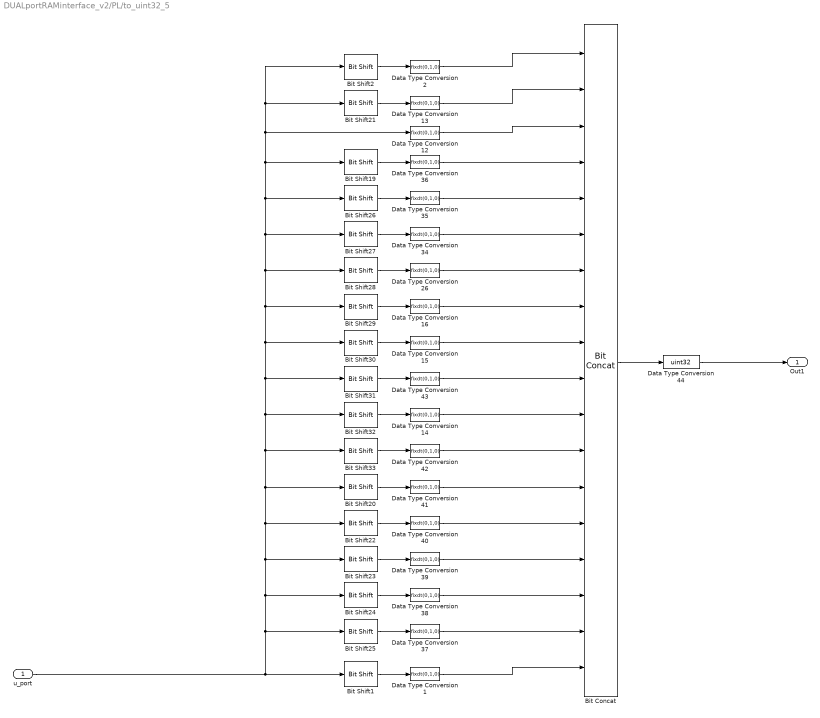
== system DUALportRAMinterface_v2/PL/to_uint32_5 ==
  u_port : Inport
  Bit Concat : hdlsllib/Logic and Bit Operations/Bit Concat  numInputs=18
  Bit Shift1 : hdlsllib/Logic and Bit Operations/Bit Shift  mode=Shift Left Logical  N=15
  Bit Shift19 : hdlsllib/Logic and Bit Operations/Bit Shift  mode=Shift Left Logical  N=1
  Bit Shift2 : hdlsllib/Logic and Bit Operations/Bit Shift  mode=Shift Right Logical  N=16
  Bit Shift20 : hdlsllib/Logic and Bit Operations/Bit Shift  mode=Shift Left Logical  N=10
  Bit Shift21 : hdlsllib/Logic and Bit Operations/Bit Shift  mode=Shift Right Logical  N=1
  Bit Shift22 : hdlsllib/Logic and Bit Operations/Bit Shift  mode=Shift Left Logical  N=11
  Bit Shift23 : hdlsllib/Logic and Bit Operations/Bit Shift  mode=Shift Left Logical  N=12
  Bit Shift24 : hdlsllib/Logic and Bit Operations/Bit Shift  mode=Shift Left Logical  N=13
  Bit Shift25 : hdlsllib/Logic and Bit Operations/Bit Shift  mode=Shift Left Logical  N=14
  Bit Shift26 : hdlsllib/Logic and Bit Operations/Bit Shift  mode=Shift Left Logical  N=2
  Bit Shift27 : hdlsllib/Logic and Bit Operations/Bit Shift  mode=Shift Left Logical  N=3
  Bit Shift28 : hdlsllib/Logic and Bit Operations/Bit Shift  mode=Shift Left Logical  N=4
  Bit Shift29 : hdlsllib/Logic and Bit Operations/Bit Shift  mode=Shift Left Logical  N=5
  Bit Shift30 : hdlsllib/Logic and Bit Operations/Bit Shift  mode=Shift Left Logical  N=6
  Bit Shift31 : hdlsllib/Logic and Bit Operations/Bit Shift  mode=Shift Left Logical  N=7
  Bit Shift32 : hdlsllib/Logic and Bit Operations/Bit Shift  mode=Shift Left Logical  N=8
  Bit Shift33 : hdlsllib/Logic and Bit Operations/Bit Shift  mode=Shift Left Logical  N=9
  Data Type Conversion{1..2,12..16,26,34..43} (18 alike) : DataTypeConversion  OutDataTypeStr=fixdt(0,1,0)  SaturateOnIntegerOverflow=off  RndMeth=Floor
  Data Type Conversion44 : DataTypeConversion  OutDataTypeStr=uint32  SaturateOnIntegerOverflow=off  RndMeth=Floor
  Out1 : Outport
  wires:
  Data Type Conversion44/1 -> Out1/1
  Data Type Conversion42/1 -> Bit Concat/12
  Bit Shift32/1 -> Data Type Conversion14/1
  Data Type Conversion40/1 -> Bit Concat/14
  Data Type Conversion37/1 -> Bit Concat/17
  Data Type Conversion38/1 -> Bit Concat/16
  Bit Shift30/1 -> Data Type Conversion15/1
  Data Type Conversion13/1 -> Bit Concat/2
  Bit Shift19/1 -> Data Type Conversion36/1
  Data Type Conversion16/1 -> Bit Concat/8
  Data Type Conversion35/1 -> Bit Concat/5
  Bit Shift1/1 -> Data Type Conversion1/1
  Bit Shift24/1 -> Data Type Conversion38/1
  Data Type Conversion36/1 -> Bit Concat/4
  Bit Shift28/1 -> Data Type Conversion26/1
  Data Type Conversion34/1 -> Bit Concat/6
  Bit Shift26/1 -> Data Type Conversion35/1
  Bit Shift29/1 -> Data Type Conversion16/1
  Bit Shift2/1 -> Data Type Conversion2/1
  Data Type Conversion41/1 -> Bit Concat/13
  Bit Shift25/1 -> Data Type Conversion37/1
  Bit Shift23/1 -> Data Type Conversion39/1
  Bit Shift33/1 -> Data Type Conversion42/1
  Data Type Conversion43/1 -> Bit Concat/10
  Data Type Conversion15/1 -> Bit Concat/9
  Data Type Conversion39/1 -> Bit Concat/15
  Bit Shift31/1 -> Data Type Conversion43/1
  Bit Shift20/1 -> Data Type Conversion41/1
  Bit Shift22/1 -> Data Type Conversion40/1
  Bit Shift27/1 -> Data Type Conversion34/1
  Data Type Conversion12/1 -> Bit Concat/3
  Bit Shift21/1 -> Data Type Conversion13/1
  Data Type Conversion26/1 -> Bit Concat/7
  Data Type Conversion2/1 -> Bit Concat/1
  Data Type Conversion1/1 -> Bit Concat/18
  Data Type Conversion14/1 -> Bit Concat/11
  u_port/1 -> Bit Shift25/1, Bit Shift24/1, Bit Shift23/1, Bit Shift22/1, Bit Shift20/1, Bit Shift33/1, Bit Shift32/1, Bit Shift31/1, Bit Shift30/1, Bit Shift29/1, Bit Shift28/1, Bit Shift27/1, Bit Shift26/1, Bit Shift19/1, Data Type Conversion12/1, Bit Shift2/1, Bit Shift21/1, Bit Shift1/1
  Bit Concat/1 -> Data Type Conversion44/1

== system DUALportRAMinterface_v2/PL/to_uint32_6 ==
  u_port : Inport
  Bit Concat : hdlsllib/Logic and Bit Operations/Bit Concat  numInputs=18
  Bit Shift1 : hdlsllib/Logic and Bit Operations/Bit Shift  mode=Shift Left Logical  N=15
  Bit Shift19 : hdlsllib/Logic and Bit Operations/Bit Shift  mode=Shift Left Logical  N=1
  Bit Shift2 : hdlsllib/Logic and Bit Operations/Bit Shift  mode=Shift Right Logical  N=16
  Bit Shift20 : hdlsllib/Logic and Bit Operations/Bit Shift  mode=Shift Left Logical  N=10
  Bit Shift21 : hdlsllib/Logic and Bit Operations/Bit Shift  mode=Shift Right Logical  N=1
  Bit Shift22 : hdlsllib/Logic and Bit Operations/Bit Shift  mode=Shift Left Logical  N=11
  Bit Shift23 : hdlsllib/Logic and Bit Operations/Bit Shift  mode=Shift Left Logical  N=12
  Bit Shift24 : hdlsllib/Logic and Bit Operations/Bit Shift  mode=Shift Left Logical  N=13
  Bit Shift25 : hdlsllib/Logic and Bit Operations/Bit Shift  mode=Shift Left Logical  N=14
  Bit Shift26 : hdlsllib/Logic and Bit Operations/Bit Shift  mode=Shift Left Logical  N=2
  Bit Shift27 : hdlsllib/Logic and Bit Operations/Bit Shift  mode=Shift Left Logical  N=3
  Bit Shift28 : hdlsllib/Logic and Bit Operations/Bit Shift  mode=Shift Left Logical  N=4
  Bit Shift29 : hdlsllib/Logic and Bit Operations/Bit Shift  mode=Shift Left Logical  N=5
  Bit Shift30 : hdlsllib/Logic and Bit Operations/Bit Shift  mode=Shift Left Logical  N=6
  Bit Shift31 : hdlsllib/Logic and Bit Operations/Bit Shift  mode=Shift Left Logical  N=7
  Bit Shift32 : hdlsllib/Logic and Bit Operations/Bit Shift  mode=Shift Left Logical  N=8
  Bit Shift33 : hdlsllib/Logic and Bit Operations/Bit Shift  mode=Shift Left Logical  N=9
  Data Type Conversion{1..2,12..16,26,34..43} (18 alike) : DataTypeConversion  OutDataTypeStr=fixdt(0,1,0)  SaturateOnIntegerOverflow=off  RndMeth=Floor
  Data Type Conversion44 : DataTypeConversion  OutDataTypeStr=uint32  SaturateOnIntegerOverflow=off  RndMeth=Floor
  Out1 : Outport
  wires:
  Bit Concat/1 -> Data Type Conversion44/1
  u_port/1 -> Bit Shift1/1, Bit Shift21/1, Bit Shift2/1, Data Type Conversion12/1, Bit Shift19/1, Bit Shift26/1, Bit Shift27/1, Bit Shift28/1, Bit Shift29/1, Bit Shift30/1, Bit Shift31/1, Bit Shift32/1, Bit Shift33/1, Bit Shift20/1, Bit Shift22/1, Bit Shift23/1, Bit Shift24/1, Bit Shift25/1
  Data Type Conversion14/1 -> Bit Concat/11
  Data Type Conversion1/1 -> Bit Concat/18
  Data Type Conversion2/1 -> Bit Concat/1
  Data Type Conversion26/1 -> Bit Concat/7
  Bit Shift21/1 -> Data Type Conversion13/1
  Data Type Conversion12/1 -> Bit Concat/3
  Bit Shift27/1 -> Data Type Conversion34/1
  Bit Shift22/1 -> Data Type Conversion40/1
  Bit Shift20/1 -> Data Type Conversion41/1
  Bit Shift31/1 -> Data Type Conversion43/1
  Data Type Conversion39/1 -> Bit Concat/15
  Data Type Conversion15/1 -> Bit Concat/9
  Data Type Conversion43/1 -> Bit Concat/10
  Bit Shift33/1 -> Data Type Conversion42/1
  Bit Shift23/1 -> Data Type Conversion39/1
  Bit Shift25/1 -> Data Type Conversion37/1
  Data Type Conversion41/1 -> Bit Concat/13
  Bit Shift2/1 -> Data Type Conversion2/1
  Bit Shift29/1 -> Data Type Conversion16/1
  Bit Shift26/1 -> Data Type Conversion35/1
  Data Type Conversion34/1 -> Bit Concat/6
  Bit Shift28/1 -> Data Type Conversion26/1
  Data Type Conversion36/1 -> Bit Concat/4
  Bit Shift24/1 -> Data Type Conversion38/1
  Bit Shift1/1 -> Data Type Conversion1/1
  Data Type Conversion35/1 -> Bit Concat/5
  Data Type Conversion16/1 -> Bit Concat/8
  Bit Shift19/1 -> Data Type Conversion36/1
  Data Type Conversion13/1 -> Bit Concat/2
  Bit Shift30/1 -> Data Type Conversion15/1
  Data Type Conversion38/1 -> Bit Concat/16
  Data Type Conversion37/1 -> Bit Concat/17
  Data Type Conversion40/1 -> Bit Concat/14
  Bit Shift32/1 -> Data Type Conversion14/1
  Data Type Conversion42/1 -> Bit Concat/12
  Data Type Conversion44/1 -> Out1/1

== system DUALportRAMinterface_v2/PL/integration_block1/D2 ==
  GAerror : Inport
  push_individual : Inport  Port=2
  reset_D2 : Inport  Port=3
  Individual_input : Inport  Port=4
  Demux : Demux  Outputs=7
  Product{,1..5} (6 alike) : Product  OutDataTypeStr=fixdt(1, 64, 32)
  Terminator : Terminator
  denom_acc11 : Sum  Inputs=+-  OutDataTypeStr=fixdt(1, 64, 32)  AccumDataTypeStr=fixdt(1, 64, 32)  SampleTime=7.50007500075001e-06
  denom_acc2 : Sum  Inputs=+-  OutDataTypeStr=fixdt(1, 64, 32)  AccumDataTypeStr=fixdt(1, 64, 32)  SampleTime=7.50007500075001e-06
  denom_acc3 : Sum  Inputs=+-  OutDataTypeStr=fixdt(1, 64, 32)  AccumDataTypeStr=fixdt(1, 64, 32)  SampleTime=7.50007500075001e-06
  individual1 : Subsystem
  output_cast1 : hdlmdlgenlib/Buffer
  reset_sw{,1..6} (7 alike) : Switch  Criteria=u2 > Threshold  SaturateOnIntegerOverflow=off  InputSameDT=off
  s_nume_acc11 : Sum  OutDataTypeStr=fixdt(1, 64, 32)  SampleTime=7.50007500075001e-06
  s_nume_acc2 : Sum  OutDataTypeStr=fixdt(1, 64, 32)  SampleTime=7.50007500075001e-06
  s_nume_acc3 : Sum  OutDataTypeStr=fixdt(1, 14, 12)  SampleTime=7.50007500075001e-06
  s_state_out11 : UnitDelay  InitialCondition="fi(0,1,64,32,\"hex\",\"0000000000000000\")"  SampleTime=7.50007500075001e-06
  s_state_out2 : UnitDelay  InitialCondition="fi(0,1,64,32,\"hex\",\"0000000000000000\")"  SampleTime=7.50007500075001e-06
  s_state_out3 : UnitDelay  InitialCondition="fi(0,1,64,32,\"hex\",\"0000000000000000\")"  SampleTime=7.50007500075001e-06
  zero{,1..6} (7 alike) : Constant  Value=0  OutDataTypeStr=fixdt(1,64,32)  SampleTime=Ts
  response : Outport
  wires:
  s_state_out11/1 -> Product5/1, Product2/1, s_state_out2/1
  s_state_out2/1 -> Product4/1, Product1/1, s_state_out3/1
  s_state_out3/1 -> Product3/1, Product/1
  Product4/1 -> reset_sw1/3
  Product1/1 -> reset_sw5/3
  s_nume_acc2/1 -> s_nume_acc3/1
  s_nume_acc11/1 -> s_nume_acc2/1
  Product5/1 -> reset_sw/3
  denom_acc2/1 -> denom_acc3/1
  Product/1 -> reset_sw4/3
  output_cast1/1 -> response/1
  denom_acc3/1 -> reset_sw3/3, s_state_out11/1
  GAerror/1 -> denom_acc11/1
  denom_acc11/1 -> denom_acc2/1
  s_nume_acc3/1 -> output_cast1/1
  Product2/1 -> reset_sw6/3
  Product3/1 -> reset_sw2/3
  individual1/7(b4) -> Product/2
  individual1/6(b3) -> Product1/2
  individual1/5(b2) -> Product2/2
  individual1/4(a4) -> Product3/2
  individual1/3(a3) -> Product4/2
  individual1/2(a2) -> Product5/2
  Demux/1 -> individual1/1(reg_in)
  Demux/3 -> individual1/3(reg_in2)
  Demux/5 -> individual1/5(reg_in4)
  Demux/2 -> individual1/2(reg_in1)
  Demux/6 -> individual1/6(reg_in5)
  Demux/4 -> individual1/4(reg_in3)
  Individual_input/1 -> Demux/1
  individual1/1(score) -> Terminator/1
  Demux/7 -> individual1/7(reg_in6)
  push_individual/1 -> individual1/8(enable)
  reset_sw/1 -> s_nume_acc11/2
  reset_D2/1 -> reset_sw6/2, reset_sw5/2, reset_sw4/2, reset_sw3/2, reset_sw/2, reset_sw2/2, reset_sw1/2
  zero/1 -> reset_sw/1
  reset_sw1/1 -> s_nume_acc2/2
  zero1/1 -> reset_sw1/1
  zero2/1 -> reset_sw2/1
  reset_sw2/1 -> s_nume_acc3/2
  reset_sw3/1 -> s_nume_acc11/1
  zero3/1 -> reset_sw3/1
  reset_sw4/1 -> denom_acc3/2
  reset_sw5/1 -> denom_acc2/2
  reset_sw6/1 -> denom_acc11/2
  zero4/1 -> reset_sw6/1
  zero5/1 -> reset_sw5/1
  zero6/1 -> reset_sw4/1
